simulink model "Commander_Stabilizer_Qdrone_wTrajTEMP"  (R2019a)
settings: Solver=ode2  StartTime=0.0  StopTime=inf  FixedStep=0.001  RelTol=1e-3  EnableMultiTasking=on
InitFcn:
  | set_param(gcs, 'ZoomFactor','FitSystem')
model workspace (MAT data in the model file):
  target_system = 1
undefined symbols (not defined in the file or in its folder): acc_calib, HIL
libraries: quarc_library x50, simulink x20, control_library x13, estimation_library x7
(part 2 of 3)

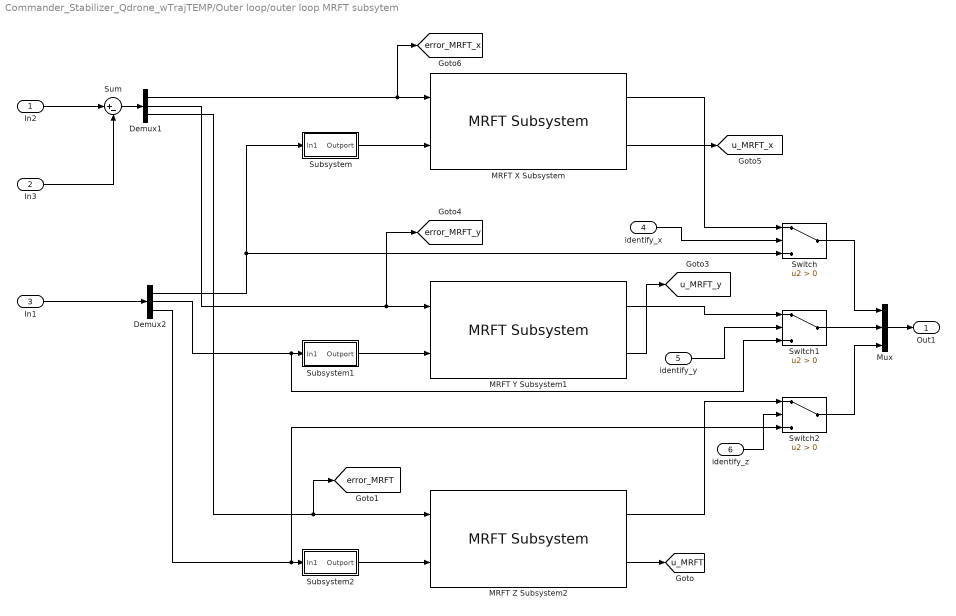
== system Commander_Stabilizer_Qdrone_wTrajTEMP/Outer loop/outer loop MRFT subsytem ==
  In2 : Inport
  In3 : Inport  Port=2
  In1 : Inport  Port=3
  identify_x : Inport  Port=4
  "identify_y " : Inport  Port=5
  identify_z : Inport  Port=6
  Demux1 : Demux  Outputs=3
  Demux2 : Demux  Outputs=3
  MRFT X Subsystem : control_library/MRFT Subsystem  h_relay=3  beta=-0.6914
  MRFT Y Subsystem1 : control_library/MRFT Subsystem  h_relay=.5  beta=-0.6914
  MRFT Z Subsystem2 : control_library/MRFT Subsystem  h_relay=3  beta=-0.73
  Mux : Mux  Inputs=3
  Subsystem : Subsystem
  Subsystem1 : Subsystem
  Subsystem2 : Subsystem
  Sum : Sum  Inputs=|+-
  Switch : Switch  Criteria=u2 > Threshold
  Switch1 : Switch  Criteria=u2 > Threshold
  Switch2 : Switch  Criteria=u2 > Threshold
  Out1 : Outport
  tag scope: error_MRFT=global, error_MRFT_x=global, error_MRFT_y=global, u_MRFT=global, u_MRFT_x=global, u_MRFT_y=global
  wires:
  In1/1 -> Demux2/1
  In2/1 -> Sum/1
  In3/1 -> Sum/2
  Sum/1 -> Demux1/1
  Demux1/1 -> [error_MRFT_x], MRFT X Subsystem/1
  Demux2/1 -> Subsystem/1(In1), Switch/3
  identify_x/1 -> Switch/2
  MRFT X Subsystem/1 -> Switch/1
  Mux/1 -> Out1/1
  Switch/1 -> Mux/1
  Subsystem/1(Outport) -> MRFT X Subsystem/2
  MRFT Y Subsystem1/1 -> Switch1/1
  MRFT Z Subsystem2/1 -> Switch2/1
  Subsystem1/1(Outport) -> MRFT Y Subsystem1/2
  Demux2/2 -> Switch1/3, Subsystem1/1(In1)
  Demux2/3 -> Switch2/3, Subsystem2/1(In1)
  Demux1/2 -> [error_MRFT_y], MRFT Y Subsystem1/1
  Demux1/3 -> MRFT Z Subsystem2/1, [error_MRFT]
  Subsystem2/1(Outport) -> MRFT Z Subsystem2/2
  Switch1/1 -> Mux/2
  Switch2/1 -> Mux/3
  "identify_y "/1 -> Switch1/2
  identify_z/1 -> Switch2/2
  MRFT Z Subsystem2/2 -> [u_MRFT]
  MRFT X Subsystem/2 -> [u_MRFT_x]
  MRFT Y Subsystem1/2 -> [u_MRFT_y]

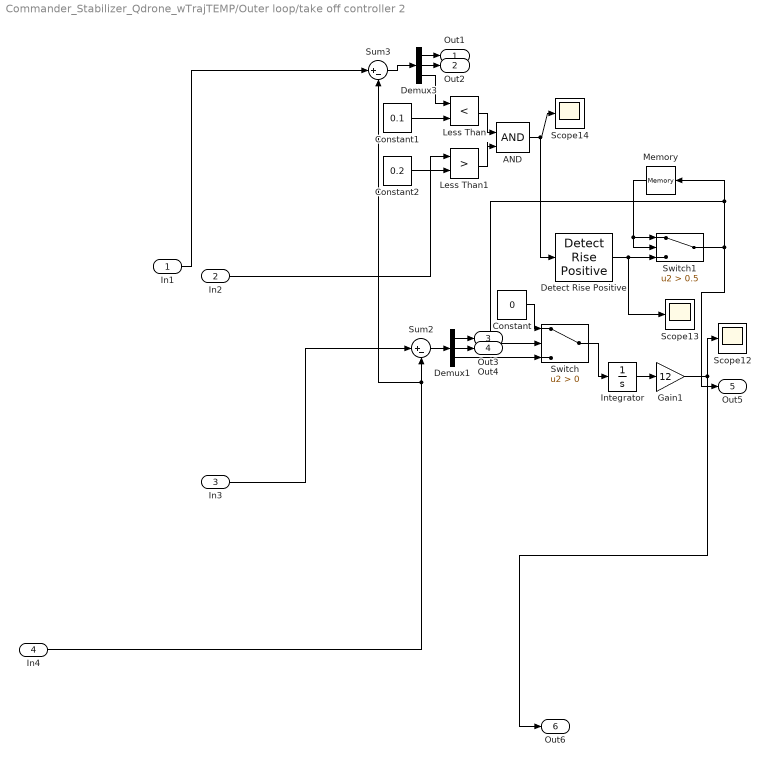
== system Commander_Stabilizer_Qdrone_wTrajTEMP/Outer loop/take off controller 2 ==
  In1 : Inport
  In2 : Inport  Port=2
  In3 : Inport  Port=3
  In4 : Inport  Port=4
  AND : Logic  IconShape=distinctive  AllPortsSameDT=off  OutDataTypeStr=boolean
  Constant : Constant  Value=0
  Constant1 : Constant  Value=0.1
  Constant2 : Constant  Value=0.2
  Demux1 : Demux  Outputs=3
  Demux3 : Demux  Outputs=3
  Detect Rise Positive : simulink/Logic and Bit Operations/Detect Rise Positive  vinit=0  OutDataTypeStr=boolean
  Gain1 : Gain  Gain=12
  Integrator : Integrator
  Less Than : RelationalOperator  Operator=<  OutDataTypeStr=boolean  RndMeth=Simplest
  Less Than1 : RelationalOperator  Operator=>  OutDataTypeStr=boolean  RndMeth=Simplest
  Memory : Memory  InitialCondition=-1
  Scope12 : Scope
  Scope13 : Scope
  Scope14 : Scope
  Sum2 : Sum  Inputs=|+-
  Sum3 : Sum  Inputs=|+-
  Switch : Switch  Criteria=u2 > Threshold
  Switch1 : Switch  Criteria=u2 > Threshold  Threshold=0.5
  Out1 : Outport
  Out2 : Outport  Port=2
  Out3 : Outport  Port=3
  Out4 : Outport  Port=4
  Out5 : Outport  Port=5
  Out6 : Outport  Port=6
  wires:
  In2/1 -> Less Than1/1
  Demux1/3 -> Switch/3
  Switch/1 -> Integrator/1
  In4/1 -> Sum3/2, Sum2/2
  Constant/1 -> Switch/1
  Sum2/1 -> Demux1/1
  Detect Rise Positive/1 -> Scope13/1, Switch1/3
  Memory/1 -> Switch1/2, Switch1/1
  Switch1/1 -> Out5/1, Switch/2, Memory/1
  Less Than1/1 -> AND/2
  Constant1/1 -> Less Than/2
  Gain1/1 -> Out6/1, Scope12/1
  Integrator/1 -> Gain1/1
  Demux1/2 -> Out4/1
  Demux3/2 -> Out2/1
  AND/1 -> Detect Rise Positive/1, Scope14/1
  Constant2/1 -> Less Than1/2
  Sum3/1 -> Demux3/1
  Less Than/1 -> AND/1
  Demux3/3 -> Less Than/1
  Demux1/1 -> Out3/1
  Demux3/1 -> Out1/1
  In3/1 -> Sum2/1
  In1/1 -> Sum3/1

== system Commander_Stabilizer_Qdrone_wTrajTEMP/log /BLACKBOX ==
  FSM Monitor Log : Inport
  Estimator log : Inport  Port=2
  Controller Log : Inport  Port=3
  MRFT info : Inport  Port=4
  Mux : Mux
  To Host File : quarc_library/Sinks/To Host/To Host File  file_name=saved_data/%m/MRFT_Commander_%{date}_%{time}.mat  variable_name=commander_data  decimation=1  sample_time=-1  file_format=MAT-file v.5  options=No header or footer  append=off  final_file_name=saved_data/Commander_Stabilizer_Qdrone_wTrajTEMP/MRFT_Commander_30-Mar-2021_18-25-03.mat  bitrate=2000000
  wires:
  Mux/1 -> To Host File/1
  FSM Monitor Log/1 -> Mux/1
  Controller Log/1 -> Mux/3
  MRFT info/1 -> Mux/4
  Estimator log/1 -> Mux/2

== system Commander_Stabilizer_Qdrone_wTrajTEMP/log /BLACKBOX1 ==
  Safety Log : Inport
  DAQ log : Inport  Port=2
  Controller log : Inport  Port=3
  motor log : Inport  Port=4
  MRFT log : Inport  Port=5
  Mux : Mux  Inputs=5
  To Host File : quarc_library/Sinks/To Host/To Host File  file_name=saved_data/%m/MRFT_Stabilizer_%{date}_%{time}.mat  variable_name=stabilizer_data  decimation=1  sample_time=-1  file_format=MAT-file v.5  options=No header or footer  append=off  final_file_name=saved_data/Commander_Stabilizer_Qdrone_wTrajTEMP/MRFT_Stabilizer_30-Mar-2021_18-25-03.mat  bitrate=2000000
      settings: SourceProductName=The database C:\Users\user\AppData\Roaming\MathWorks\MATLAB\R2017a\slblocks_master.db is locked, or a table in the database is locked. (database is locked)
  wires:
  Mux/1 -> To Host File/1
  Safety Log/1 -> Mux/1
  DAQ log/1 -> Mux/2
  Controller log/1 -> Mux/3
  MRFT log/1 -> Mux/5
  motor log/1 -> Mux/4

== system Commander_Stabilizer_Qdrone_wTrajTEMP/log /Inner loop MRFT ==
  Gain : Gain  ParamDataTypeStr=double
  Gain1 : Gain  ParamDataTypeStr=double
  Mux2 : Mux  Inputs=10
  Sample Time : quarc_library/Sources/Time/Sample Time  Priority=-99  sample_time=qc_get_step_size
      settings: SourceProductName=The database C:\Users\user\AppData\Roaming\MathWorks\MATLAB\R2017a\slblocks_master.db is locked, or a table in the database is locked. (database is locked)
  Out1 : Outport
  wires:
  Gain/1 -> Mux2/2
  Gain1/1 -> Mux2/5
  [pitch_MRFT_MODE] -> Gain1/1
  Sample Time/1 -> Mux2/1
  [roll_error_MRFT] -> Mux2/4
  [roll_MRFT_MODE] -> Gain/1
  [pitch_mrft_output] -> Mux2/6
  [pitch_error_MRFT] -> Mux2/7
  [roll_mrft_output] -> Mux2/3
  Mux2/1 -> Out1/1
  [yaw_MRFT_MODE] -> Mux2/8
  [yaw_mrft_output] -> Mux2/9
  [yaw_error_MRFT] -> Mux2/10

== system Commander_Stabilizer_Qdrone_wTrajTEMP/log /MRFT data concat  ==
  Gain : Gain  ParamDataTypeStr=double
  Gain1 : Gain  ParamDataTypeStr=double
  Gain4 : Gain  ParamDataTypeStr=double
  Mux2 : Mux  Inputs=10
  Sample Time : quarc_library/Sources/Time/Sample Time  Priority=-99  sample_time=qc_get_step_size
      settings: SourceProductName=The database C:\Users\user\AppData\Roaming\MathWorks\MATLAB\R2017a\slblocks_master.db is locked, or a table in the database is locked. (database is locked)
  Out1 : Outport
  wires:
  [MRFT_PID_MODE_y] -> Gain1/1
  Gain1/1 -> Mux2/5
  [MRFT_PID_MODE_z] -> Gain/1
  Gain/1 -> Mux2/2
  [error_MRFT] -> Mux2/4
  Sample Time/1 -> Mux2/1
  [u_MRFT_y] -> Mux2/6
  [error_MRFT_y] -> Mux2/7
  [u_MRFT] -> Mux2/3
  Mux2/1 -> Out1/1
  [MRFT_PID_MODE_x] -> Gain4/1
  Gain4/1 -> Mux2/8
  [u_MRFT_x] -> Mux2/9
  [error_MRFT_x] -> Mux2/10

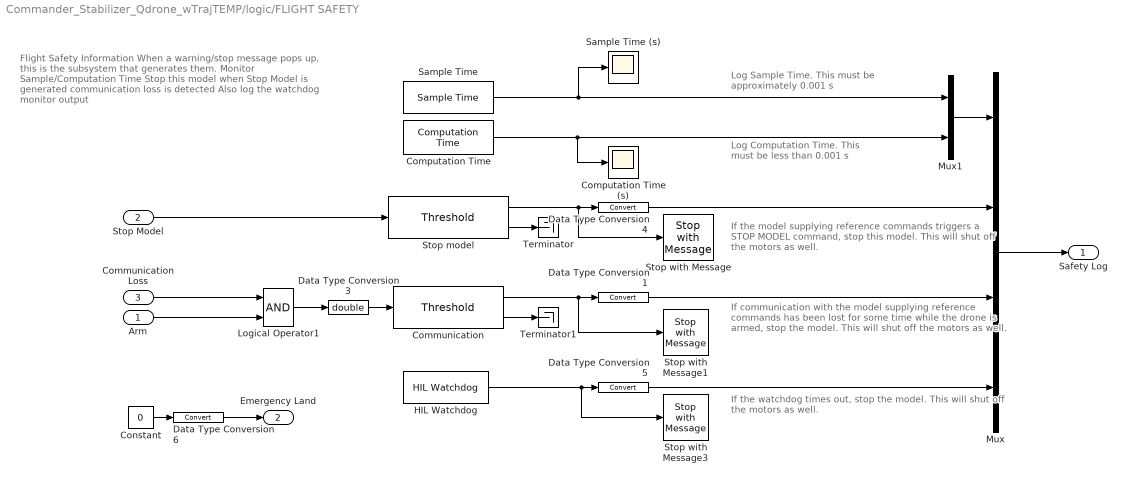
== system Commander_Stabilizer_Qdrone_wTrajTEMP/logic/FLIGHT SAFETY ==
  note: Flight Safety Information
      |
      | When a warning/stop message pops up, this is the subsystem
      | that generates them.
      |
      | Monitor Sample/Computation Time
      | Stop this model
      | when Stop Model is generated
      | communication loss is detected
      | Also log the watchdog monitor output
  note: Log Sample Time. This must be approximately 0.001 s
  note: Log Computation Time. This must be less than 0.001 s
  note: If the model supplying reference commands triggers a STOP MODEL command, stop this model. This will shut off the motors as well.
  note: If communication with the model supplying reference commands has been lost for some time while the drone is armed, stop the model. This will shut off the motors as well.
  note: If the watchdog times out, stop the model. This will shut off the motors as well.
  Arm : Inport
  Stop Model : Inport  Port=2
  Communication Loss : Inport  Port=3
  Communication : quarc_library/Discontinuities/Threshold  operator=>=  param_src=Specify via dialog  threshold=0.5  duration=1
      settings: SourceProductName=The database C:\Users\user\AppData\Roaming\MathWorks\MATLAB\R2017a\slblocks_master.db is locked, or a table in the database is locked. (database is locked)
  Computation Time : quarc_library/Sources/Time/Computation Time  sample_time=qc_get_step_size  use_model=on  use_cpu_time=off
      settings: SourceProductName=The database C:\Users\user\AppData\Roaming\MathWorks\MATLAB\R2017a\slblocks_master.db is locked, or a table in the database is locked. (database is locked)
  Computation Time (s) : Scope
  Constant : Constant  Value=0
  Data Type Conversion{1,4..6} (4 alike) : DataTypeConversion
  Data Type Conversion3 : DataTypeConversion  OutDataTypeStr=double
  HIL Watchdog : quarc_library/Data Acquisition/Generic/Watchdog/HIL Watchdog  object_name=HIL-1  timeout=0.1  sample_time=qc_get_step_size  active=off
      settings: AttributesFormatString=(%<object_name>)  SourceProductName=QUARC Targets
  Logical Operator1 : Logic  AllPortsSameDT=off  OutDataTypeStr=boolean
  Mux : Mux
  Mux1 : Mux  Inputs=2
  Sample Time : quarc_library/Sources/Time/Sample Time  Priority=-99  sample_time=qc_get_step_size
      settings: SourceProductName=The database C:\Users\user\AppData\Roaming\MathWorks\MATLAB\R2017a\slblocks_master.db is locked, or a table in the database is locked. (database is locked)
  Sample Time (s) : Scope
  Stop model : quarc_library/Discontinuities/Threshold  operator=>=  param_src=Specify via dialog  threshold=0.5  duration=0.1
      settings: SourceProductName=The database C:\Users\user\AppData\Roaming\MathWorks\MATLAB\R2017a\slblocks_master.db is locked, or a table in the database is locked. (database is locked)
  Stop with Message : quarc_library/Sinks/Error Handling/Stop with Message  message_type=Fixed error message  message_icon=Information  message=QDrone Stabilizer: Commander Terminated
      settings: SourceProductName=The database C:\Users\user\AppData\Roaming\MathWorks\MATLAB\R2017a\slblocks_master.db is locked, or a table in the database is locked. (database is locked)
  Stop with Message1 : quarc_library/Sinks/Error Handling/Stop with Message  message_type=Fixed error message  message_icon=Warning  message=QDrone Stabilizer: Communication with Commander lost
      settings: SourceProductName=The database C:\Users\user\AppData\Roaming\MathWorks\MATLAB\R2017a\slblocks_master.db is locked, or a table in the database is locked. (database is locked)
  Stop with Message3 : quarc_library/Sinks/Error Handling/Stop with Message  message_type=Fixed error message  message_icon=Information  message=QDrone Stabilizer: HIL Watchdog timer expired
      settings: SourceProductName=The database C:\Users\user\AppData\Roaming\MathWorks\MATLAB\R2017a\slblocks_master.db is locked, or a table in the database is locked. (database is locked)
  Terminator : Terminator
  Terminator1 : Terminator
  Safety Log : Outport
  Emergency Land : Outport  Port=2
  wires:
  Mux/1 -> Safety Log/1
  Computation Time/1 -> Computation Time (s)/1, Mux1/2
  Sample Time/1 -> Sample Time (s)/1, Mux1/1
  Data Type Conversion4/1 -> Mux/2
  HIL Watchdog/1 -> Stop with Message3/1, Data Type Conversion5/1
  Stop model/2 -> Terminator/1
  Stop model/1 -> Data Type Conversion4/1, Stop with Message/1
  Stop Model/1 -> Stop model/1
  Communication/2 -> Terminator1/1
  Logical Operator1/1 -> Data Type Conversion3/1
  Data Type Conversion1/1 -> Mux/3
  Arm/1 -> Logical Operator1/2
  Communication/1 -> Data Type Conversion1/1, Stop with Message1/1
  Data Type Conversion3/1 -> Communication/1
  Communication Loss/1 -> Logical Operator1/1
  Mux1/1 -> Mux/1
  Constant/1 -> Data Type Conversion6/1
  Data Type Conversion6/1 -> Emergency Land/1
  Data Type Conversion5/1 -> Mux/4

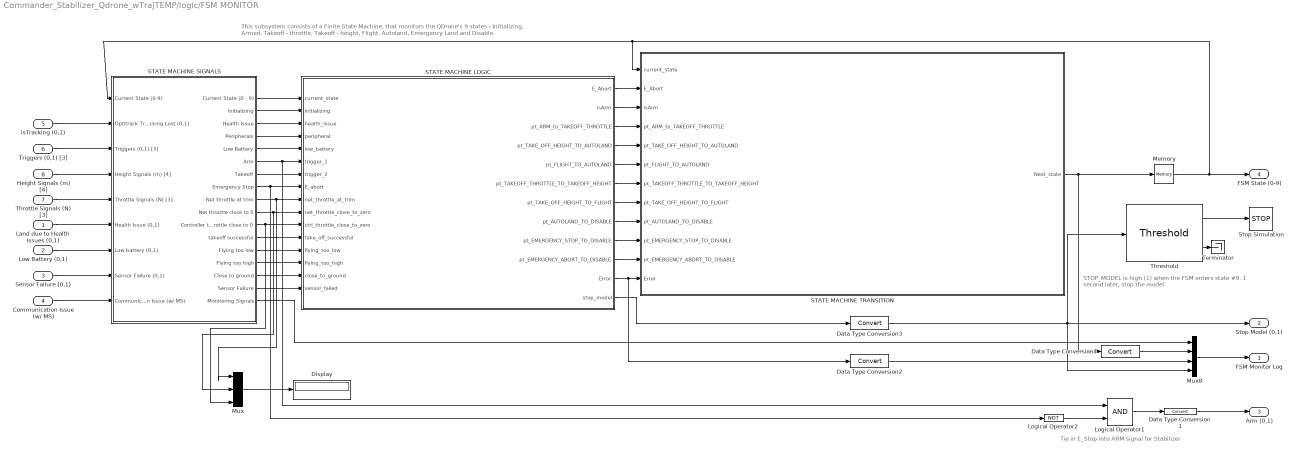
== system Commander_Stabilizer_Qdrone_wTrajTEMP/logic/FSM MONITOR ==
  note: This subsystem consists of a Finite State Machine, that monitors the QDrone's 9 states - Initializing, Armed, Takeoff - throttle, Takeoff - height, Flight, Autoland, Emergency Land and Disable.
  note: Tie in E_Stop into ARM signal for Stabilizer
  note: STOP_MODEL is high (1) when the FSM enters state #9.
      | 1 second later, stop the model.
  Land due to Health Issues (0,1) : Inport
  Low Battery (0,1) : Inport  Port=2
  Sensor Failure (0,1) : Inport  Port=3
  Communication Issue (w/ MS) : Inport  Port=4
  isTracking (0,1) : Inport  Port=5
  Triggers (0,1) [3] : Inport  Port=6
  Throttle Signals (N) [3] : Inport  Port=7
  Height Signals (m) [4] : Inport  Port=8
  Data Type Conversion{1..4} (4 alike) : DataTypeConversion
  Display : Display
  Logical Operator1 : Logic  AllPortsSameDT=off  OutDataTypeStr=boolean
  Logical Operator2 : Logic  Operator=NOT  AllPortsSameDT=off  OutDataTypeStr=boolean
  Memory : Memory  InitialCondition=1
  Mux : Mux  Inputs=3
  Mux8 : Mux  Inputs=[17 1 1 1]
  STATE MACHINE LOGIC : MATLAB Function  TreatAsAtomicUnit=on
  STATE MACHINE SIGNALS : Subsystem
  STATE MACHINE TRANSITION : MATLAB Function  TreatAsAtomicUnit=on
  Stop Simulation : Stop
  Terminator : Terminator
  Threshold : quarc_library/Discontinuities/Threshold  operator=>=  param_src=Specify via dialog  threshold=0.5  duration=1
      settings: SourceProductName=QUARC Targets
  FSM Monitor Log : Outport
  Stop Model (0,1) : Outport  Port=2
  Arm (0,1) : Outport  Port=3
  FSM State (0-9) : Outport  Port=4
  wires:
  STATE MACHINE LOGIC/1(E_Abort) -> STATE MACHINE TRANSITION/2(E_Abort)
  STATE MACHINE LOGIC/11(Error) -> STATE MACHINE TRANSITION/12(Error), Data Type Conversion2/1
  STATE MACHINE LOGIC/6(pt_TAKEOFF_THROTTLE_TO_TAKEOFF_HEIGHT) -> STATE MACHINE TRANSITION/7(pt_TAKEOFF_THROTTLE_TO_TAKEOFF_HEIGHT)
  STATE MACHINE LOGIC/7(pt_TAKE_OFF_HEIGHT_TO_FLIGHT) -> STATE MACHINE TRANSITION/8(pt_TAKE_OFF_HEIGHT_TO_FLIGHT)
  STATE MACHINE LOGIC/8(pt_AUTOLAND_TO_DISABLE) -> STATE MACHINE TRANSITION/9(pt_AUTOLAND_TO_DISABLE)
  STATE MACHINE LOGIC/9(pt_EMERGENCY_STOP_TO_DISABLE) -> STATE MACHINE TRANSITION/10(pt_EMERGENCY_STOP_TO_DISABLE)
  STATE MACHINE LOGIC/10(pt_EMERGENCY_ABORT_TO_DISABLE) -> STATE MACHINE TRANSITION/11(pt_EMERGENCY_ABORT_TO_DISABLE)
  STATE MACHINE SIGNALS/2(Initializing) -> STATE MACHINE LOGIC/2(initializing)
  STATE MACHINE SIGNALS/3(Health Issue) -> STATE MACHINE LOGIC/3(health_issue)
  STATE MACHINE SIGNALS/4(Peripherals) -> STATE MACHINE LOGIC/4(peripheral)
  STATE MACHINE SIGNALS/5(Low Battery) -> STATE MACHINE LOGIC/5(low_battery)
  STATE MACHINE SIGNALS/7(Takeoff) -> STATE MACHINE LOGIC/7(trigger_2)
  STATE MACHINE SIGNALS/9(Net throttle at trim) -> Mux/1, STATE MACHINE LOGIC/9(net_throttle_at_trim)
  STATE MACHINE SIGNALS/10(Net throttle close to 0) -> Mux/2, STATE MACHINE LOGIC/10(net_throttle_close_to_zero)
  STATE MACHINE SIGNALS/11(Controller throttle close to 0) -> Mux/3, STATE MACHINE LOGIC/11(ctrl_throttle_close_to_zero)
  STATE MACHINE SIGNALS/12(takeoff successful) -> STATE MACHINE LOGIC/12(take_off_successful)
  STATE MACHINE SIGNALS/13(Flying too low) -> STATE MACHINE LOGIC/13(flying_too_low)
  STATE MACHINE SIGNALS/14(Flying too high) -> STATE MACHINE LOGIC/14(flying_too_high)
  STATE MACHINE SIGNALS/15(Close to ground) -> STATE MACHINE LOGIC/15(close_to_ground)
  STATE MACHINE TRANSITION/1(Next_state) -> Data Type Conversion4/1, Memory/1
  Mux8/1 -> FSM Monitor Log/1
  STATE MACHINE SIGNALS/1("Current State (0 - 9)  ") -> STATE MACHINE LOGIC/1(current_state)
  STATE MACHINE SIGNALS/16("  Sensor Failure") -> STATE MACHINE LOGIC/16(sensor_failed)
  STATE MACHINE SIGNALS/17(Monitoring Signals) -> Mux8/1
  Sensor Failure (0,1)/1 -> STATE MACHINE SIGNALS/8(Sensor Failure (0,1))
  Low Battery (0,1)/1 -> STATE MACHINE SIGNALS/7(Low battery (0,1))
  Land due to Health Issues (0,1)/1 -> STATE MACHINE SIGNALS/6("Health Issue (0,1)  ")
  Data Type Conversion1/1 -> Arm (0,1)/1
  Logical Operator1/1 -> Data Type Conversion1/1
  STATE MACHINE SIGNALS/8(Emergency Stop) -> Logical Operator2/1, STATE MACHINE LOGIC/8(E_abort)
  Logical Operator2/1 -> Logical Operator1/2
  STATE MACHINE SIGNALS/6(Arm) -> Logical Operator1/1, STATE MACHINE LOGIC/6(trigger_1)
  Triggers (0,1) [3]/1 -> STATE MACHINE SIGNALS/3(Triggers (0,1) [3])
  Communication Issue (w/ MS)/1 -> STATE MACHINE SIGNALS/9(Communication Issue (w/ MS))
  isTracking (0,1)/1 -> STATE MACHINE SIGNALS/2("Optitrack Tracking Lost (0,1)  ")
  Data Type Conversion2/1 -> Mux8/3
  Data Type Conversion4/1 -> Mux8/2
  Throttle Signals (N) [3]/1 -> STATE MACHINE SIGNALS/5(Throttle Signals (N) [3])
  Height Signals (m) [4]/1 -> STATE MACHINE SIGNALS/4(Height Signals (m) [4])
  Threshold/2 -> Terminator/1
  Data Type Conversion3/1 -> Threshold/1, Stop Model (0,1)/1, Mux8/4
  Threshold/1 -> Stop Simulation/1
  Memory/1 -> FSM State (0-9)/1, STATE MACHINE TRANSITION/1(current_state), STATE MACHINE SIGNALS/1(Current State (0-9))
  STATE MACHINE LOGIC/2(isArm) -> STATE MACHINE TRANSITION/3(isArm)
  STATE MACHINE LOGIC/3(pt_ARM_to_TAKEOFF_THROTTLE) -> STATE MACHINE TRANSITION/4(pt_ARM_to_TAKEOFF_THROTTLE)
  STATE MACHINE LOGIC/4(pt_TAKE_OFF_HEIGHT_TO_AUTOLAND) -> STATE MACHINE TRANSITION/5(pt_TAKE_OFF_HEIGHT_TO_AUTOLAND)
  STATE MACHINE LOGIC/5(pt_FLIGHT_TO_AUTOLAND) -> STATE MACHINE TRANSITION/6(pt_FLIGHT_TO_AUTOLAND)
  STATE MACHINE LOGIC/12(stop_model) -> Data Type Conversion3/1
  Mux/1 -> Display/1

== system Commander_Stabilizer_Qdrone_wTrajTEMP/motor command mapper/Set commands ==
  note: Write to motors and LEDs
  Motor Cmd (%) [4] : Inport
  Arm (0,1) : Inport  Port=2
  low battery : Inport  Port=3
  Bias - Pulse Offset (%) : Bias  Bias=125e-6
  HIL Write : quarc_library/Data Acquisition/Generic/Immediate I//O/HIL Write  object_name=HIL-1  analog_channels=[]  pwm_channels=[0:3]  digital_channels=[5:7 9:23]  other_channels=[]  sample_time=-1  active=off  vector_input=on
      settings: SourceProductName=The database C:\Users\user\AppData\Roaming\MathWorks\MATLAB\R2017a\slblocks_master.db is locked, or a table in the database is locked. (database is locked)
  Percent to quarter : Gain  Gain=125e-6
  Product : Product
  Red - Low Voltage Green - Armed Blue - Disarmed : Subsystem
  wires:
  Bias - Pulse Offset (%)/1 -> HIL Write/1
  Percent to quarter/1 -> Bias - Pulse Offset (%)/1
  Motor Cmd (%) [4]/1 -> Product/1
  Product/1 -> Percent to quarter/1
  Red - Low Voltage Green - Armed Blue - Disarmed/1(LEDs (%) [18]) -> HIL Write/2
  Arm (0,1)/1 -> Product/2, Red - Low Voltage Green - Armed Blue - Disarmed/1(Arm (0,1))
  low battery/1 -> Red - Low Voltage Green - Armed Blue - Disarmed/2(Low Battery (0,1))

== system Commander_Stabilizer_Qdrone_wTrajTEMP/DAQ /Sensor Failure Monitoring/Sensor Failure (Accelerometer) ==
  note: Check for flat-line ZERO Accelerometer data (no data)
  Sensor Input : Inport
  Clock : Clock
  Compare To Constant : simulink/Logic and Bit Operations/Compare To Constant  relop=>=  const=1  OutDataTypeStr=boolean
  Demux1 : Demux  Outputs=3
  Logical Operator : Logic  Operator=OR  Inputs=3  AllPortsSameDT=off  OutDataTypeStr=boolean
  Logical Operator1 : Logic  AllPortsSameDT=off  OutDataTypeStr=boolean
  Terminator1 : Terminator
  Terminator3 : Terminator
  Terminator4 : Terminator
  Threshold : quarc_library/Discontinuities/Threshold  operator===  param_src=Specify via dialog  threshold=0  duration=1
      settings: SourceProductName=The database C:\Users\user\AppData\Roaming\MathWorks\MATLAB\R2017a\slblocks_master.db is locked, or a table in the database is locked. (database is locked)
  Threshold1 : quarc_library/Discontinuities/Threshold  operator===  param_src=Specify via dialog  threshold=0  duration=1
      settings: SourceProductName=The database C:\Users\user\AppData\Roaming\MathWorks\MATLAB\R2017a\slblocks_master.db is locked, or a table in the database is locked. (database is locked)
  Threshold2 : quarc_library/Discontinuities/Threshold  operator===  param_src=Specify via dialog  threshold=0  duration=1
      settings: SourceProductName=The database C:\Users\user\AppData\Roaming\MathWorks\MATLAB\R2017a\slblocks_master.db is locked, or a table in the database is locked. (database is locked)
  Sensor Fault : Outport
  wires:
  Threshold/2 -> Terminator1/1
  Threshold1/2 -> Terminator3/1
  Logical Operator/1 -> Logical Operator1/2
  Demux1/2 -> Threshold1/1
  Demux1/3 -> Threshold2/1
  Demux1/1 -> Threshold/1
  Threshold2/1 -> Logical Operator/3
  Threshold2/2 -> Terminator4/1
  Sensor Input/1 -> Demux1/1
  Logical Operator1/1 -> Sensor Fault/1
  Compare To Constant/1 -> Logical Operator1/1
  Threshold1/1 -> Logical Operator/2
  Threshold/1 -> Logical Operator/1
  Clock/1 -> Compare To Constant/1

== system Commander_Stabilizer_Qdrone_wTrajTEMP/DAQ /Sensor Failure Monitoring/Sensor Failure (Gyroscope) ==
  note: Check for flat-line ZERO Gyro data (no data)
  Sensor Input : Inport
  Clock : Clock
  Compare To Constant : simulink/Logic and Bit Operations/Compare To Constant  relop=>=  const=1  OutDataTypeStr=boolean
  Demux1 : Demux  Outputs=3
  Logical Operator : Logic  Operator=OR  Inputs=3  AllPortsSameDT=off  OutDataTypeStr=boolean
  Logical Operator1 : Logic  AllPortsSameDT=off  OutDataTypeStr=boolean
  Terminator1 : Terminator
  Terminator3 : Terminator
  Terminator4 : Terminator
  Threshold : quarc_library/Discontinuities/Threshold  operator===  param_src=Specify via dialog  threshold=0  duration=1
      settings: SourceProductName=The database C:\Users\user\AppData\Roaming\MathWorks\MATLAB\R2017a\slblocks_master.db is locked, or a table in the database is locked. (database is locked)
  Threshold1 : quarc_library/Discontinuities/Threshold  operator===  param_src=Specify via dialog  threshold=0  duration=1
      settings: SourceProductName=The database C:\Users\user\AppData\Roaming\MathWorks\MATLAB\R2017a\slblocks_master.db is locked, or a table in the database is locked. (database is locked)
  Threshold2 : quarc_library/Discontinuities/Threshold  operator===  param_src=Specify via dialog  threshold=0  duration=1
      settings: SourceProductName=The database C:\Users\user\AppData\Roaming\MathWorks\MATLAB\R2017a\slblocks_master.db is locked, or a table in the database is locked. (database is locked)
  Sensor Fault : Outport
  wires:
  Clock/1 -> Compare To Constant/1
  Threshold/1 -> Logical Operator/1
  Threshold1/1 -> Logical Operator/2
  Compare To Constant/1 -> Logical Operator1/1
  Logical Operator1/1 -> Sensor Fault/1
  Sensor Input/1 -> Demux1/1
  Threshold2/2 -> Terminator4/1
  Threshold2/1 -> Logical Operator/3
  Demux1/1 -> Threshold/1
  Demux1/3 -> Threshold2/1
  Demux1/2 -> Threshold1/1
  Logical Operator/1 -> Logical Operator1/2
  Threshold1/2 -> Terminator3/1
  Threshold/2 -> Terminator1/1

== system Commander_Stabilizer_Qdrone_wTrajTEMP/Inner loop controller /inner loop MRFT subsytem/MRFT_NEW  ==
  Error : Inport
  Clock1 : Clock
  Constant5 : Constant  Value=-0.737
  Constant6 : Constant  Value=0.3
  Constant7 : Constant  Value=0.001
  Constant9 : Constant  Value=10
  MATLAB Function : MATLAB Function  TreatAsAtomicUnit=on  SystemSampleTime=0.001
  Scope2 : Scope  NumInputPorts=6
  control output : Outport
  wires:
  MATLAB Function/4(sw_max_o) -> Scope2/5
  MATLAB Function/2(e_max_o) -> Scope2/2
  Constant7/1 -> MATLAB Function/4(no_switch_delay_in_s)
  Clock1/1 -> MATLAB Function/6(sim_time)
  MATLAB Function/3(e_min_o) -> Scope2/3
  MATLAB Function/5(sw_min_o) -> Scope2/6
  Constant5/1 -> MATLAB Function/2(beta)
  Error/1 -> Scope2/4, MATLAB Function/1(err)
  Constant9/1 -> MATLAB Function/5(num_of_peak_conf_samples)
  Constant6/1 -> MATLAB Function/3(h)
  MATLAB Function/1(output) -> control output/1, Scope2/1  "control output"

== system Commander_Stabilizer_Qdrone_wTrajTEMP/Inner loop controller /inner loop MRFT subsytem/MRFT_NEW 1 ==
  Error : Inport
  Clock1 : Clock
  Constant5 : Constant  Value=-0.737
  Constant6 : Constant  Value=0.3
  Constant7 : Constant  Value=0.001
  Constant9 : Constant  Value=10
  MATLAB Function : MATLAB Function  TreatAsAtomicUnit=on  SystemSampleTime=0.001
  Scope2 : Scope  NumInputPorts=6
  control output : Outport
  wires:
  MATLAB Function/4(sw_max_o) -> Scope2/5
  MATLAB Function/2(e_max_o) -> Scope2/2
  Constant7/1 -> MATLAB Function/4(no_switch_delay_in_s)
  Clock1/1 -> MATLAB Function/6(sim_time)
  MATLAB Function/3(e_min_o) -> Scope2/3
  MATLAB Function/5(sw_min_o) -> Scope2/6
  Constant5/1 -> MATLAB Function/2(beta)
  Error/1 -> Scope2/4, MATLAB Function/1(err)
  Constant9/1 -> MATLAB Function/5(num_of_peak_conf_samples)
  Constant6/1 -> MATLAB Function/3(h)
  MATLAB Function/1(output) -> control output/1, Scope2/1  "control output"

== system Commander_Stabilizer_Qdrone_wTrajTEMP/Inner loop controller /inner loop MRFT subsytem/MRFT_input ==
  data : Inport
  switch : Inport  Port=2
  Constant : Constant  Value=0
  Switch : Switch  Criteria=u2 > Threshold  Threshold=.5
  Out1 : Outport
  wires:
  Constant/1 -> Switch/3
  Switch/1 -> Out1/1
  data/1 -> Switch/1
  switch/1 -> Switch/2

== system Commander_Stabilizer_Qdrone_wTrajTEMP/Inner loop controller /inner loop MRFT subsytem/MRFT_input1 ==
  data : Inport
  switch : Inport  Port=2
  Constant : Constant  Value=0
  Switch : Switch  Criteria=u2 > Threshold  Threshold=.5
  Out1 : Outport
  wires:
  Constant/1 -> Switch/3
  Switch/1 -> Out1/1
  data/1 -> Switch/1
  switch/1 -> Switch/2

== system Commander_Stabilizer_Qdrone_wTrajTEMP/Inner loop controller /inner loop MRFT subsytem/Subsystem ==
  In1 : Inport
  Logical Operator1 : Logic  Operator=OR  AllPortsSameDT=off  OutDataTypeStr=boolean
  Logical Operator2 : Logic  Commented=on  Operator=NOT  AllPortsSameDT=off  OutDataTypeStr=boolean
  MRFT1 : From  Commented=on  GotoTag=takeoff_cmd  TagVisibility=global
  Memory : Memory
  Switch1 : Switch  Criteria=u2 > Threshold  Threshold=0.5
  low Pass Filter : TransferFcn  Numerator=[pi/3]  Denominator=[1 pi/3]
  Outport : Outport
  tag scope: filter_PID_roll=global
  wires:
  In1/1 -> Switch1/3
  MRFT1/1 -> Logical Operator2/1
  low Pass Filter/1 -> Outport/1, [filter_PID_roll]
  Logical Operator1/1 -> Switch1/2
  Memory/1 -> Switch1/1
  Logical Operator2/1 -> Logical Operator1/1
  [roll_MRFT_MODE] -> Logical Operator1/2
  [filter_PID_roll] -> Memory/1
  Switch1/1 -> low Pass Filter/1

== system Commander_Stabilizer_Qdrone_wTrajTEMP/Inner loop controller /inner loop MRFT subsytem/Subsystem1 ==
  In1 : Inport
  Logical Operator1 : Logic  Operator=OR  AllPortsSameDT=off  OutDataTypeStr=boolean
  Logical Operator2 : Logic  Commented=on  Operator=NOT  AllPortsSameDT=off  OutDataTypeStr=boolean
  MRFT1 : From  Commented=on  GotoTag=takeoff_cmd  TagVisibility=global
  Memory : Memory
  Switch1 : Switch  Criteria=u2 > Threshold  Threshold=0.5
  low Pass Filter : TransferFcn  Numerator=[pi/3]  Denominator=[1 pi/3]
  Outport : Outport
  tag scope: filter_PID_pitch=global
  wires:
  Switch1/1 -> low Pass Filter/1
  [filter_PID_pitch] -> Memory/1
  [pitch_MRFT_MODE] -> Logical Operator1/2
  Logical Operator2/1 -> Logical Operator1/1
  Memory/1 -> Switch1/1
  Logical Operator1/1 -> Switch1/2
  low Pass Filter/1 -> [filter_PID_pitch], Outport/1
  MRFT1/1 -> Logical Operator2/1
  In1/1 -> Switch1/3

== system Commander_Stabilizer_Qdrone_wTrajTEMP/Inner loop controller /inner loop MRFT subsytem/Subsystem2 ==
  In1 : Inport
  Logical Operator1 : Logic  Operator=OR  AllPortsSameDT=off  OutDataTypeStr=boolean
  Logical Operator2 : Logic  Commented=on  Operator=NOT  AllPortsSameDT=off  OutDataTypeStr=boolean
  MRFT1 : From  Commented=on  GotoTag=takeoff_cmd  TagVisibility=global
  Memory : Memory
  Switch1 : Switch  Criteria=u2 > Threshold  Threshold=0.5
  low Pass Filter : TransferFcn  Numerator=[pi/3]  Denominator=[1 pi/3]
  Outport : Outport
  tag scope: filter_PID_yaw=global
  wires:
  In1/1 -> Switch1/3
  MRFT1/1 -> Logical Operator2/1
  low Pass Filter/1 -> Outport/1, [filter_PID_yaw]
  Logical Operator1/1 -> Switch1/2
  Memory/1 -> Switch1/1
  Logical Operator2/1 -> Logical Operator1/1
  [yaw_MRFT_MODE] -> Logical Operator1/2
  [filter_PID_yaw] -> Memory/1
  Switch1/1 -> low Pass Filter/1

== system Commander_Stabilizer_Qdrone_wTrajTEMP/Outer loop/outer loop MRFT subsytem/Subsystem ==
  In1 : Inport
  Logical Operator1 : Logic  Operator=OR  AllPortsSameDT=off  OutDataTypeStr=boolean
  Logical Operator2 : Logic  Commented=on  Operator=NOT  AllPortsSameDT=off  OutDataTypeStr=boolean
  MRFT1 : From  Commented=on  GotoTag=takeoff_cmd  TagVisibility=global
  Memory : Memory
  Switch1 : Switch  Criteria=u2 > Threshold  Threshold=0.5
  low Pass Filter : TransferFcn  Numerator=[pi]  Denominator=[1 pi]
  Outport : Outport
  tag scope: filter_PID_thrust_x=global
  wires:
  In1/1 -> Switch1/3
  MRFT1/1 -> Logical Operator2/1
  low Pass Filter/1 -> Outport/1, [filter_PID_thrust_x]
  Logical Operator1/1 -> Switch1/2
  Memory/1 -> Switch1/1
  Logical Operator2/1 -> Logical Operator1/1
  [MRFT_PID_MODE_x] -> Logical Operator1/2
  [filter_PID_thrust_x] -> Memory/1
  Switch1/1 -> low Pass Filter/1

== system Commander_Stabilizer_Qdrone_wTrajTEMP/Outer loop/outer loop MRFT subsytem/Subsystem1 ==
  In1 : Inport
  Logical Operator1 : Logic  Operator=OR  AllPortsSameDT=off  OutDataTypeStr=boolean
  Logical Operator2 : Logic  Commented=on  Operator=NOT  AllPortsSameDT=off  OutDataTypeStr=boolean
  MRFT1 : From  Commented=on  GotoTag=takeoff_cmd  TagVisibility=global
  Memory : Memory
  Switch1 : Switch  Criteria=u2 > Threshold  Threshold=0.5
  low Pass Filter : TransferFcn  Numerator=[pi]  Denominator=[1 pi]
  Outport : Outport
  tag scope: filter_PID_thrust_y=global
  wires:
  Switch1/1 -> low Pass Filter/1
  [filter_PID_thrust_y] -> Memory/1
  [MRFT_PID_MODE_y] -> Logical Operator1/2
  Logical Operator2/1 -> Logical Operator1/1
  Memory/1 -> Switch1/1
  Logical Operator1/1 -> Switch1/2
  low Pass Filter/1 -> [filter_PID_thrust_y], Outport/1
  MRFT1/1 -> Logical Operator2/1
  In1/1 -> Switch1/3

== system Commander_Stabilizer_Qdrone_wTrajTEMP/Outer loop/outer loop MRFT subsytem/Subsystem2 ==
  In1 : Inport
  Logical Operator1 : Logic  Operator=OR  AllPortsSameDT=off  OutDataTypeStr=boolean
  Logical Operator2 : Logic  Commented=on  Operator=NOT  AllPortsSameDT=off  OutDataTypeStr=boolean
  MRFT1 : From  Commented=on  GotoTag=takeoff_cmd  TagVisibility=global
  Memory : Memory
  Switch1 : Switch  Criteria=u2 > Threshold  Threshold=0.5
  low Pass Filter : TransferFcn  Numerator=[pi]  Denominator=[1 pi]
  Outport : Outport
  tag scope: filter_PID_thrust_z=global
  wires:
  In1/1 -> Switch1/3
  MRFT1/1 -> Logical Operator2/1
  low Pass Filter/1 -> Outport/1, [filter_PID_thrust_z]
  Logical Operator1/1 -> Switch1/2
  Memory/1 -> Switch1/1
  Logical Operator2/1 -> Logical Operator1/1
  [MRFT_PID_MODE_z] -> Logical Operator1/2
  [filter_PID_thrust_z] -> Memory/1
  Switch1/1 -> low Pass Filter/1

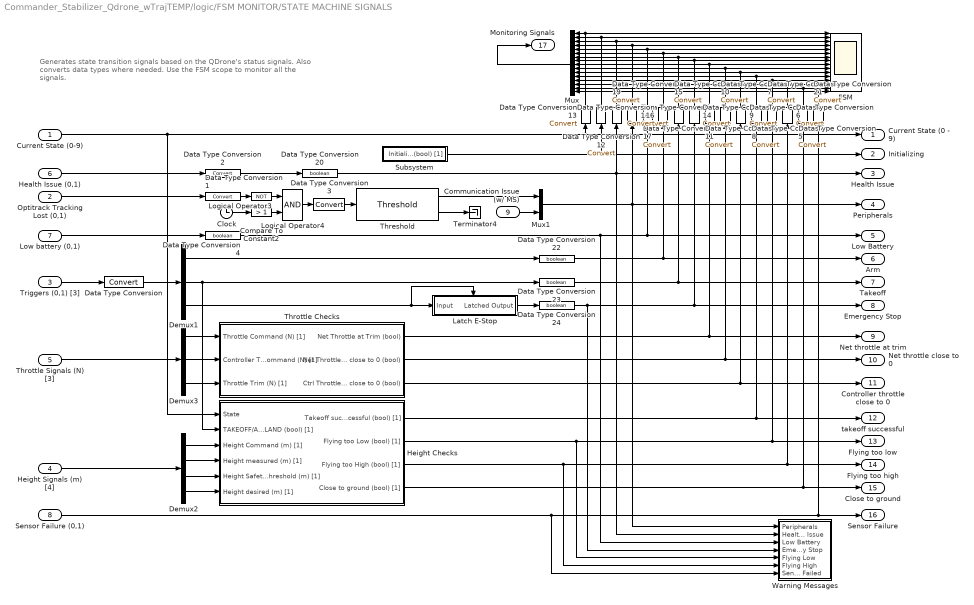
== system Commander_Stabilizer_Qdrone_wTrajTEMP/logic/FSM MONITOR/STATE MACHINE SIGNALS ==
  note: Generates state transition signals based on the QDrone's status signals.
      | Also converts data types where needed.
      |
      | Use the FSM scope to monitor all the signals.
  Current State (0-9) : Inport
  "Optitrack Tracking Lost (0,1)  " : Inport  Port=2
  Triggers (0,1) [3] : Inport  Port=3
  Height Signals (m) [4] : Inport  Port=4
  Throttle Signals (N) [3] : Inport  Port=5
  "Health Issue (0,1)  " : Inport  Port=6
  Low battery (0,1) : Inport  Port=7
  Sensor Failure (0,1) : Inport  Port=8
  Communication Issue (w/ MS) : Inport  Port=9
  Clock : Clock
  Compare To Constant2 : simulink/Logic and Bit Operations/Compare To Constant  relop=>  const=1  OutDataTypeStr=boolean
  Data Type Conversion{,1..3,5..19,21} (20 alike) : DataTypeConversion
  Data Type Conversion{4,20,22..24} (5 alike) : DataTypeConversion  OutDataTypeStr=boolean
  Demux1 : Demux  Outputs=3
  Demux2 : Demux
  Demux3 : Demux  Outputs=3
  FSM : Scope  NumInputPorts=16
  Height Checks : Subsystem
  Latch E-Stop : Subsystem  TreatAsAtomicUnit=on
  Logical Operator3 : Logic  Operator=NOT  AllPortsSameDT=off  OutDataTypeStr=boolean
  Logical Operator4 : Logic  AllPortsSameDT=off  OutDataTypeStr=boolean
  Mux : Mux  Inputs=16
  Mux1 : Mux  Inputs=2
  Subsystem : Subsystem
  Terminator4 : Terminator
  Threshold : quarc_library/Discontinuities/Threshold  operator=>=  param_src=Specify via dialog  threshold=0.5  duration=0.2
      settings: SourceProductName=QUARC Targets
  Throttle Checks : Subsystem
  Warning Messages : Subsystem
  "Current State (0 - 9)  " : Outport
  Initializing : Outport  Port=2
  Health Issue : Outport  Port=3
  Peripherals : Outport  Port=4
  Low Battery : Outport  Port=5
  Arm : Outport  Port=6
  Takeoff : Outport  Port=7
  Emergency Stop : Outport  Port=8
  Net throttle at trim : Outport  Port=9
  Net throttle close to 0 : Outport  Port=10
  Controller throttle close to 0 : Outport  Port=11
  takeoff successful : Outport  Port=12
  Flying too low : Outport  Port=13
  Flying too high : Outport  Port=14
  Close to ground : Outport  Port=15
  "  Sensor Failure" : Outport  Port=16
  Monitoring Signals : Outport  Port=17
  wires:
  Triggers (0,1) [3]/1 -> Data Type Conversion/1
  Demux2/1 -> Height Checks/3(Height Command (m) [1])
  Demux3/1 -> Throttle Checks/1(Throttle Command (N) [1])
  Height Signals (m) [4]/1 -> Demux2/1
  Demux2/4 -> Height Checks/6(Height desired (m) [1])
  Throttle Signals (N) [3]/1 -> Demux3/1
  Throttle Checks/3(Ctrl Throttle close to 0 (bool)) -> Data Type Conversion9/1, Controller throttle close to 0/1
  Demux1/1 -> Data Type Conversion22/1
  Throttle Checks/2(Net Throttle close to 0 (bool)) -> Data Type Conversion10/1, Net throttle close to 0/1
  Height Checks/1(Takeoff successful (bool) [1]) -> Data Type Conversion8/1, takeoff successful/1
  Demux2/3 -> Height Checks/5(Height Safety Threshold (m) [1])
  Demux1/2 -> Height Checks/2(TAKEOFF/AUTOLAND (bool) [1]), Data Type Conversion23/1
  Demux2/2 -> Height Checks/4(Height measured (m) [1])
  Demux3/2 -> Throttle Checks/2(Controller Throttle Command (N) [1])
  Demux3/3 -> Throttle Checks/3(Throttle Trim (N) [1])
  Throttle Checks/1(Net Throttle at Trim (bool)) -> Data Type Conversion11/1, Net throttle at trim/1
  Height Checks/3(Flying too High (bool) [1]) -> Warning Messages/6(Flying High), Data Type Conversion6/1, Flying too high/1
  Height Checks/4(Close to ground (bool) [1]) -> Data Type Conversion5/1, Close to ground/1
  Data Type Conversion/1 -> Demux1/1
  "Health Issue (0,1)  "/1 -> Data Type Conversion2/1
  Low battery (0,1)/1 -> Data Type Conversion4/1
  Height Checks/2(Flying too Low (bool) [1]) -> Warning Messages/5(Flying Low), Data Type Conversion7/1, Flying too low/1
  Sensor Failure (0,1)/1 -> Data Type Conversion21/1, "  Sensor Failure"/1, Warning Messages/7(Sensor Failed)
  Mux1/1 -> Data Type Conversion18/1, Warning Messages/1(Peripherals), Peripherals/1
  Subsystem/1(Initializing (bool) [1]) -> Data Type Conversion12/1, Initializing/1
  Communication Issue (w/ MS)/1 -> Mux1/2
  Data Type Conversion1/1 -> Logical Operator3/1
  Data Type Conversion3/1 -> Threshold/1
  Compare To Constant2/1 -> Logical Operator4/2
  Clock/1 -> Compare To Constant2/1
  Logical Operator4/1 -> Data Type Conversion3/1
  Threshold/2 -> Terminator4/1
  Logical Operator3/1 -> Logical Operator4/1
  Threshold/1 -> Mux1/1
  "Optitrack Tracking Lost (0,1)  "/1 -> Data Type Conversion1/1
  Current State (0-9)/1 -> Data Type Conversion13/1, "Current State (0 - 9)  "/1, Height Checks/1(State)
  Data Type Conversion2/1 -> Data Type Conversion20/1
  Data Type Conversion4/1 -> Warning Messages/3(Low Battery), Data Type Conversion17/1, Low Battery/1
  Mux/1 -> Monitoring Signals/1
  Data Type Conversion13/1 -> Mux/1, FSM/1
  Data Type Conversion12/1 -> Mux/2, FSM/2
  Data Type Conversion19/1 -> Mux/3, FSM/3
  Data Type Conversion18/1 -> Mux/4, FSM/4
  Data Type Conversion17/1 -> Mux/5, FSM/5
  Data Type Conversion16/1 -> Mux/6, FSM/6
  Data Type Conversion15/1 -> Mux/7, FSM/7
  Data Type Conversion14/1 -> Mux/8, FSM/8
  Data Type Conversion11/1 -> Mux/9, FSM/9
  Data Type Conversion10/1 -> Mux/10, FSM/10
  Data Type Conversion9/1 -> Mux/11, FSM/11
  Data Type Conversion8/1 -> Mux/12, FSM/12
  Data Type Conversion7/1 -> Mux/13, FSM/13
  Data Type Conversion6/1 -> Mux/14, FSM/14
  Data Type Conversion5/1 -> FSM/15, Mux/15
  Data Type Conversion21/1 -> FSM/16, Mux/16
  Data Type Conversion20/1 -> Data Type Conversion19/1, Warning Messages/2(Health Issue), Health Issue/1
  Data Type Conversion22/1 -> Data Type Conversion16/1, Arm/1
  Data Type Conversion23/1 -> Data Type Conversion15/1, Takeoff/1
  Data Type Conversion24/1 -> Warning Messages/4("Emergency Stop "), Data Type Conversion14/1, Emergency Stop/1
  Latch E-Stop/1(Latched Output) -> Data Type Conversion24/1
  Demux1/3 -> Latch E-Stop/Trigger, Latch E-Stop/1(Input)

== system Commander_Stabilizer_Qdrone_wTrajTEMP/motor command mapper/Set commands/Red - Low Voltage Green - Armed Blue - Disarmed ==
  note: PCB LED 3
  note: PCB LED 2
  note: PCB LED 1
  note: PCB LED 5
  note: PCB LED 4
  note: Onboard LED
  Arm (0,1) : Inport
  Low Battery (0,1) : Inport  Port=2
  Blue : Constant  Value=[0 0 1]
  Green : Constant  Value=[0 1 0]
  MATLAB Function LED Color Assignment : MATLAB Function  TreatAsAtomicUnit=on
  Multiport Switch : MultiPortSwitch
  Mux : Mux  Inputs=[3 3 3 3 3 3]
  Red : Constant  Value=[1 0 0]
  LEDs (%) [18] : Outport
  wires:
  Multiport Switch/1 -> Mux/4, Mux/5, Mux/6, Mux/3, Mux/2, Mux/1
  Red/1 -> Multiport Switch/2
  Green/1 -> Multiport Switch/3
  Blue/1 -> Multiport Switch/4
  Arm (0,1)/1 -> MATLAB Function LED Color Assignment/1(arm)
  MATLAB Function LED Color Assignment/1(value) -> Multiport Switch/1
  Low Battery (0,1)/1 -> MATLAB Function LED Color Assignment/2(low_battery)
  Mux/1 -> LEDs (%) [18]/1

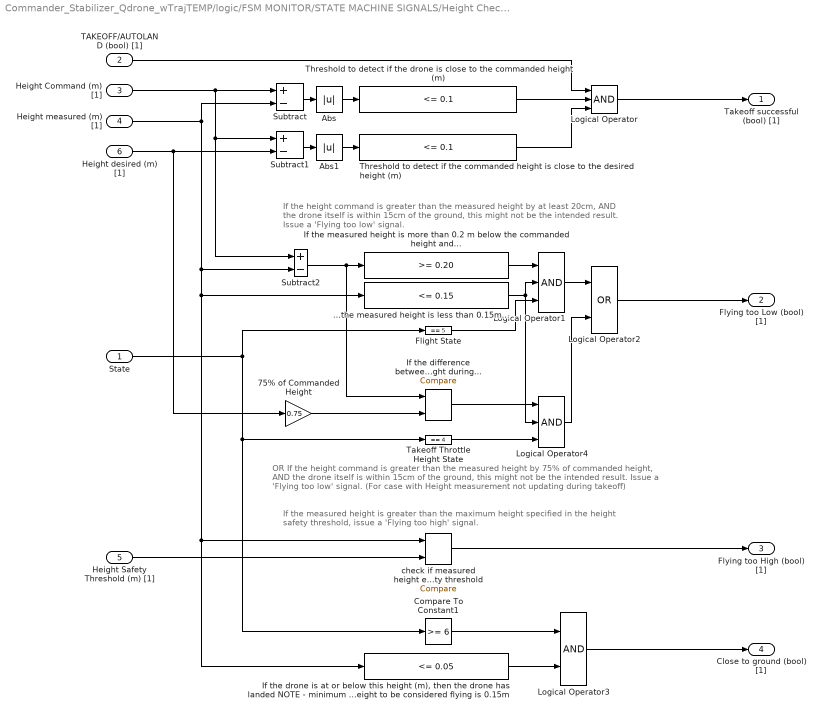
== system Commander_Stabilizer_Qdrone_wTrajTEMP/logic/FSM MONITOR/STATE MACHINE SIGNALS/Height Checks ==
  note: If the height command is greater than the measured height by at least 20cm, AND the drone itself is
      | within 15cm of the ground, this might not be the intended result. Issue a 'Flying too low' signal.
  note: If the measured height is greater than the maximum height specified in the height safety threshold,
      | issue a 'Flying too high' signal.
  note: OR If the height command is greater than the measured height by 75% of commanded height, AND
      | the drone itself is within 15cm of the ground, this might not be the intended result. Issue a 'Flying too low' signal.
      | (For case with Height measurement not updating during takeoff)
  State : Inport
  TAKEOFF/AUTOLAND (bool) [1] : Inport  Port=2
  Height Command (m) [1] : Inport  Port=3
  Height measured (m) [1] : Inport  Port=4
  Height Safety Threshold (m) [1] : Inport  Port=5
  Height desired (m) [1] : Inport  Port=6
  ...the measured height is less than 0.15m... : simulink/Logic and Bit Operations/Compare To Constant  relop=<=  const=0.15  OutDataTypeStr=boolean
  75% of Commanded Height : Gain  Gain=0.75
  Abs : Abs
  Abs1 : Abs
  Compare To Constant1 : simulink/Logic and Bit Operations/Compare To Constant  relop=>=  const=6  OutDataTypeStr=boolean
  Flight State : simulink/Logic and Bit Operations/Compare To Constant  relop===  const=5  OutDataTypeStr=boolean
  If the difference between the measured and commanded height is greater than 75% of the commanded height during... : quarc_library/Logic Operations/Compare  operator=>=  output_data_type=boolean
      settings: SourceProductName=QUARC Targets
  "If the drone is at or below this height (m), then the drone has landed NOTE - minimum height to be considered flying is 0.15m   " : simulink/Logic and Bit Operations/Compare To Constant  relop=<=  const=0.05  OutDataTypeStr=boolean
  If the measured height is more than 0.2 m below the commanded height and... : simulink/Logic and Bit Operations/Compare To Constant  relop=>=  const=0.20  OutDataTypeStr=boolean
  Logical Operator : Logic  Inputs=3  AllPortsSameDT=off  OutDataTypeStr=boolean
  Logical Operator1 : Logic  Inputs=3  AllPortsSameDT=off  OutDataTypeStr=boolean
  Logical Operator2 : Logic  Operator=OR  AllPortsSameDT=off  OutDataTypeStr=boolean
  Logical Operator3 : Logic  AllPortsSameDT=off  OutDataTypeStr=boolean
  Logical Operator4 : Logic  Inputs=3  AllPortsSameDT=off  OutDataTypeStr=boolean
  Subtract : Sum  Inputs=+-
  Subtract1 : Sum  Inputs=+-
  Subtract2 : Sum  Inputs=+-
  Takeoff Throttle Height State : simulink/Logic and Bit Operations/Compare To Constant  relop===  const=4  OutDataTypeStr=boolean
  Threshold to detect if the commanded height is close to the desired height (m) : simulink/Logic and Bit Operations/Compare To Constant  relop=<=  const=0.1  OutDataTypeStr=boolean
  Threshold to detect if the drone is close to the commanded height (m) : simulink/Logic and Bit Operations/Compare To Constant  relop=<=  const=0.1  OutDataTypeStr=boolean
  check if measured height exceeds maximum height safety threshold : quarc_library/Logic Operations/Compare  operator=>=  output_data_type=boolean
      settings: SourceProductName=QUARC Targets
  Takeoff successful (bool) [1] : Outport
  Flying too Low (bool) [1] : Outport  Port=2
  Flying too High (bool) [1] : Outport  Port=3
  Close to ground (bool) [1] : Outport  Port=4
  wires:
  Logical Operator/1 -> Takeoff successful (bool) [1]/1
  Logical Operator2/1 -> Flying too Low (bool) [1]/1
  Subtract1/1 -> Abs1/1
  Threshold to detect if the commanded height is close to the desired height (m)/1 -> Logical Operator/3
  Abs/1 -> Threshold to detect if the drone is close to the commanded height (m)/1
  Threshold to detect if the drone is close to the commanded height (m)/1 -> Logical Operator/2
  Abs1/1 -> Threshold to detect if the commanded height is close to the desired height (m)/1
  Height desired (m) [1]/1 -> 75% of Commanded Height/1, Subtract1/2
  TAKEOFF/AUTOLAND (bool) [1]/1 -> Logical Operator/1
  Subtract/1 -> Abs/1
  If the measured height is more than 0.2 m below the commanded height and.../1 -> Logical Operator1/1
  Logical Operator1/1 -> Logical Operator2/1
  Height Command (m) [1]/1 -> Subtract1/1, Subtract2/1, Subtract/1
  ...the measured height is less than 0.15m.../1 -> Logical Operator4/2, Logical Operator1/2
  check if measured height exceeds maximum height safety threshold/1 -> Flying too High (bool) [1]/1
  Height Safety Threshold (m) [1]/1 -> check if measured height exceeds maximum height safety threshold/2
  State/1 -> Takeoff Throttle Height State/1, Compare To Constant1/1, Flight State/1
  Logical Operator3/1 -> Close to ground (bool) [1]/1
  "If the drone is at or below this height (m), then the drone has landed NOTE - minimum height to be considered flying is 0.15m   "/1 -> Logical Operator3/2
  Compare To Constant1/1 -> Logical Operator3/1
  Height measured (m) [1]/1 -> Subtract/2, ...the measured height is less than 0.15m.../1, "If the drone is at or below this height (m), then the drone has landed NOTE - minimum height to be considered flying is 0.15m   "/1, check if measured height exceeds maximum height safety threshold/1, Subtract2/2
  Logical Operator4/1 -> Logical Operator2/2
  Flight State/1 -> Logical Operator1/3
  Subtract2/1 -> If the difference between the measured and commanded height is greater than 75% of the commanded height during.../1, If the measured height is more than 0.2 m below the commanded height and.../1
  If the difference between the measured and commanded height is greater than 75% of the commanded height during.../1 -> Logical Operator4/1
  Takeoff Throttle Height State/1 -> Logical Operator4/3
  75% of Commanded Height/1 -> If the difference between the measured and commanded height is greater than 75% of the commanded height during.../2

== system Commander_Stabilizer_Qdrone_wTrajTEMP/logic/FSM MONITOR/STATE MACHINE SIGNALS/Latch E-Stop ==
  Input : Inport
  Trigger : TriggerPort  VariantControl=Variant
  Latched Output : Outport  InitialOutput=0
  wires:
  Input/1 -> Latched Output/1

== system Commander_Stabilizer_Qdrone_wTrajTEMP/logic/FSM MONITOR/STATE MACHINE SIGNALS/Subsystem ==
  note: Give 2s for any bias removal/estimation/preparation
  Clock : Clock
  Compare To Constant : simulink/Logic and Bit Operations/Compare To Constant  relop=<=  const=2  OutDataTypeStr=boolean
  Initializing (bool) [1] : Outport
  wires:
  Clock/1 -> Compare To Constant/1
  Compare To Constant/1 -> Initializing (bool) [1]/1

== system Commander_Stabilizer_Qdrone_wTrajTEMP/logic/FSM MONITOR/STATE MACHINE SIGNALS/Throttle Checks ==
  Throttle Command (N) [1] : Inport
  Controller Throttle Command (N) [1] : Inport  Port=2
  Throttle Trim (N) [1] : Inport  Port=3
  Abs : Abs
  Abs1 : Abs
  Subtract : Sum  Inputs=+-
  Threshold below which throttle can be assumed to be close to zero (N) (15%) : simulink/Logic and Bit Operations/Compare To Constant  relop=<=  const=3.5  OutDataTypeStr=boolean
  Threshold to determine if the controller throttle is close to zero (N) (6%) : simulink/Logic and Bit Operations/Compare To Constant  relop=<=  const=2.40  OutDataTypeStr=boolean
  Threshold to determine if throttle is close to the trim value (N) (2.5%) : simulink/Logic and Bit Operations/Compare To Constant  relop=<=  const=0.7  OutDataTypeStr=boolean
  Net Throttle at Trim (bool) : Outport
  Net Throttle close to 0 (bool) : Outport  Port=2
  Ctrl Throttle close to 0 (bool) : Outport  Port=3
  wires:
  Throttle Command (N) [1]/1 -> Subtract/1, Threshold below which throttle can be assumed to be close to zero (N) (15%)/1
  Throttle Trim (N) [1]/1 -> Subtract/2
  Abs/1 -> Threshold to determine if throttle is close to the trim value (N) (2.5%)/1
  Subtract/1 -> Abs/1
  Threshold to determine if throttle is close to the trim value (N) (2.5%)/1 -> Net Throttle at Trim (bool)/1
  Threshold below which throttle can be assumed to be close to zero (N) (15%)/1 -> Net Throttle close to 0 (bool)/1
  Abs1/1 -> Threshold to determine if the controller throttle is close to zero (N) (6%)/1
  Controller Throttle Command (N) [1]/1 -> Abs1/1
  Threshold to determine if the controller throttle is close to zero (N) (6%)/1 -> Ctrl Throttle close to 0 (bool)/1

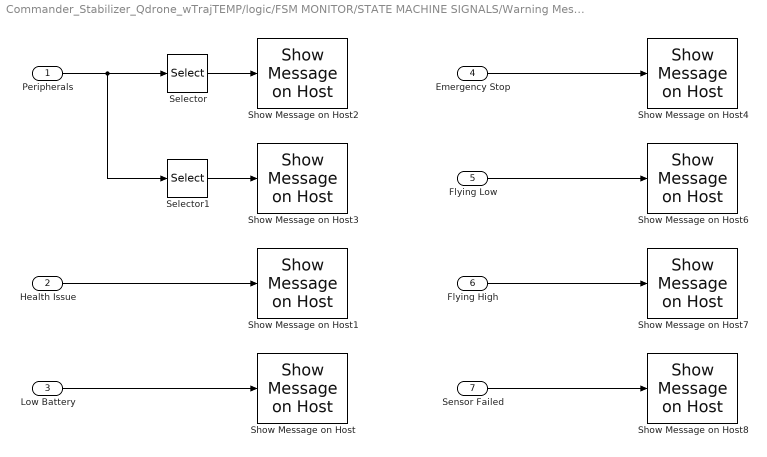
== system Commander_Stabilizer_Qdrone_wTrajTEMP/logic/FSM MONITOR/STATE MACHINE SIGNALS/Warning Messages ==
  Peripherals : Inport
  Health Issue : Inport  Port=2
  Low Battery : Inport  Port=3
  "Emergency Stop " : Inport  Port=4
  Flying Low : Inport  Port=5
  Flying High : Inport  Port=6
  Sensor Failed : Inport  Port=7
  Selector : Selector  InputPortWidth=2  IndexOptions=Index vector (dialog)  Indices=[1]  OutputSizes=1
  Selector1 : Selector  InputPortWidth=2  IndexOptions=Index vector (dialog)  Indices=[2]  OutputSizes=1
  Show Message on Host : quarc_library/Sinks/Error Handling/Show Message on Host  message_type=Fixed error message  message_icon=Warning  message=Commander: Low Battery
      settings: AttributesFormatString="\"%<message>\""  SourceProductName=QUARC Targets
  Show Message on Host1 : quarc_library/Sinks/Error Handling/Show Message on Host  message_type=Fixed error message  message_icon=Warning  message=Commander: Stabilizer not healthy (losing heartbeats!)
      settings: AttributesFormatString="\"%<message>\""  SourceProductName=QUARC Targets
  Show Message on Host2 : quarc_library/Sinks/Error Handling/Show Message on Host  message_type=Fixed error message  message_icon=Warning  message=Commander: Optitrack isn't tracking
      settings: AttributesFormatString="\"%<message>\""  SourceProductName=QUARC Targets
  Show Message on Host3 : quarc_library/Sinks/Error Handling/Show Message on Host  message_type=Fixed error message  message_icon=Warning  message=Commander: Host Stream Issue
      settings: AttributesFormatString="\"%<message>\""  SourceProductName=QUARC Targets
  Show Message on Host4 : quarc_library/Sinks/Error Handling/Show Message on Host  message_type=Fixed error message  message_icon=Warning  message=Commander: Emergency Stop Triggered
      settings: AttributesFormatString="\"%<message>\""  SourceProductName=QUARC Targets
  Show Message on Host6 : quarc_library/Sinks/Error Handling/Show Message on Host  message_type=Fixed error message  message_icon=Warning  message=Commander: Flying low
      settings: AttributesFormatString="\"%<message>\""  SourceProductName=QUARC Targets
  Show Message on Host7 : quarc_library/Sinks/Error Handling/Show Message on Host  message_type=Fixed error message  message_icon=Warning  message=Commander: Flying high
      settings: AttributesFormatString="\"%<message>\""  SourceProductName=QUARC Targets
  Show Message on Host8 : quarc_library/Sinks/Error Handling/Show Message on Host  message_type=Fixed error message  message_icon=Warning  message=Commander: Sensor Failure
      settings: AttributesFormatString="\"%<message>\""  SourceProductName=QUARC Targets
  wires:
  Selector/1 -> Show Message on Host2/1
  Selector1/1 -> Show Message on Host3/1
  Health Issue/1 -> Show Message on Host1/1
  Peripherals/1 -> Selector1/1, Selector/1
  Low Battery/1 -> Show Message on Host/1
  "Emergency Stop "/1 -> Show Message on Host4/1
  Flying Low/1 -> Show Message on Host6/1
  Flying High/1 -> Show Message on Host7/1
  Sensor Failed/1 -> Show Message on Host8/1
